simulink model "single_wheel_susp_demo"  (R2025a)
settings: Solver=VariableStepAuto  StartTime=0.0  StopTime=10.0  MaxStep=0.01  RelTol=1e-3
undefined symbols (not defined in the file or in its folder): robot, world
settings Model: Creator=yaremadzulynsky  LastModifiedBy=yaremadzulynsky

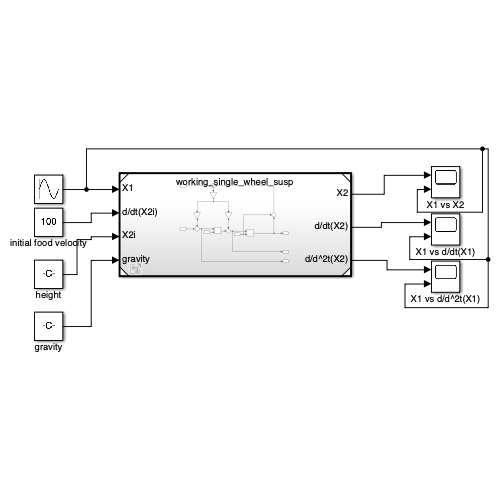
[thumbnail: Simulink's stored preview of the top-level diagram]
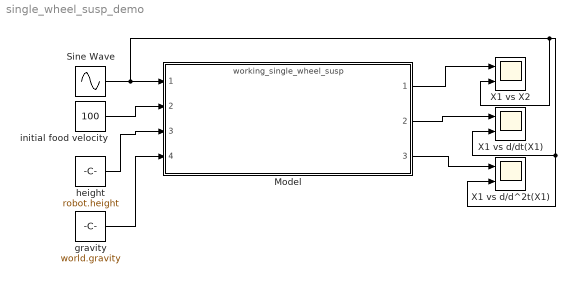
== system single_wheel_susp_demo ==
  Model : ModelReference  ModelNameDialog=working_single_wheel_susp.slx  SimulationMode=Normal  ModelReferenceVersion=1.28
  Sine Wave : Sin  Amplitude=0  Frequency=15  SampleTime=0
  X1 vs X2 : Scope  NumInputPorts=2
      settings: ActiveDisplayYMinimum=-1.6578158577365798  ActiveDisplayYMaximum=13.32179081829884
  X1 vs d/d^2t(X1) : Scope  NumInputPorts=2
      settings: ActiveDisplayYMinimum=-1.2147617693969959  ActiveDisplayYMaximum=2.1836137872966082  DataLoggingVariableName=ScopeData2
  X1 vs d/dt(X1) : Scope  NumInputPorts=2
      settings: ActiveDisplayYMinimum=-0.755362167014505  ActiveDisplayYMaximum=0.55220064527891433
  gravity : Constant  Value=world.gravity
  height : Constant  Value=robot.height
  initial food velocity : Constant  Value=100
  wires:
  Model/1 -> X1 vs X2/1
  Sine Wave/1 -> X1 vs X2/2, X1 vs d/dt(X1)/2, X1 vs d/d^2t(X1)/2, Model/1
  height/1 -> Model/3
  Model/3 -> X1 vs d/d^2t(X1)/1
  Model/2 -> X1 vs d/dt(X1)/1
  gravity/1 -> Model/4
  initial food velocity/1 -> Model/2
